simulink model "qpsk_rx_frame_sync"  (R2020a)
settings: Solver=VariableStepAuto  StartTime=0.0  StopTime=4000/3.2e6  RelTol=1e-3
PreLoadFcn:
  | setup_qpsk_receiver
InitFcn:
  | setup_qpsk_receiver
values from neighbouring files (symbols this model uses):
  tx_data = [tx_data mbuf]    [setup_receiver.m]
undefined symbols (not defined in the file or in its folder): AXI4, designMultirateFIR, Lite, xlfda_numerator
libraries: xbsIndex_r4 x244, dspmlti4 x11, hdlsllib x9, dspswit3 x4, commrandsrc3 x2, dspsigops x2, simulink x1
(part 2 of 4)

== system qpsk_rx_frame_sync/QPSK System/QPSK RX Generation ==
  Data In : Inport
  CIC Decimation : dspmlti4/CIC Decimation  filtFrom=Dialog parameters  filtobj=CICDECIM  ftype=Decimator  R=5  M=1  N=3  filterInternals=Full precision  BPS=[16 16 16 16]  FLPS=0  outputWordLength=32  outputFracLength=0  launchFVT=off  framing=Maintain input frame rate  RateOptions=Allow multirate processing
      settings: SourceProductBaseCode=DS
  FDATool : xbsIndex_r4/FDATool  block_type=fdatool
      settings: infoedit=FDATool
  FIR 0 : dspmlti4/FIR Decimation  FilterSource=Dialog parameters  h=xlfda_numerator('FDATool')  D=2  filtStruct=Direct form  FilterObject=fir0  framing=Enforce single-rate processing  inputOffset=0  outputBufInitCond=0  roundingMode=Floor  overflowMode=off  firstCoeffDataTypeStr=Inherit: Same word length as input  firstCoeffMin=[]  firstCoeffMax=[]  firstCoeffLastDataTypeStr=Inherit: Same word length as input  outputMode=Binary point scaling  outputWordLength=16  outputFracLength=14  outputDataTypeStr=fixdt(1,16,14)  outputMin=[]  outputMax=[]  outputLastDataTypeStr=fixdt(1,16,14)
  Gain : Gain  Gain=2^(floor(log2(5^3)))/(5^3)  ParamDataTypeStr=fixdt(1,16,14)  OutDataTypeStr=fixdt(1,16,14)
  RRC Receive Filter : Subsystem
  Shift Arithmetic : ArithShift  BitShiftNumber=floor(log2(5^3))  BitShiftDirection=Right
  Unbuffer : Unbuffer
  Data Out : Outport  VectorParamsAs1DForOutWhenUnconnected=off
  wires:
  RRC Receive Filter/1(Data Out) -> Data Out/1
  Gain/1 -> RRC Receive Filter/1(Data In)
  Shift Arithmetic/1 -> Gain/1
  CIC Decimation/1 -> Shift Arithmetic/1
  FIR 0/1 -> CIC Decimation/1
  Data In/1 -> Unbuffer/1
  Unbuffer/1 -> FIR 0/1

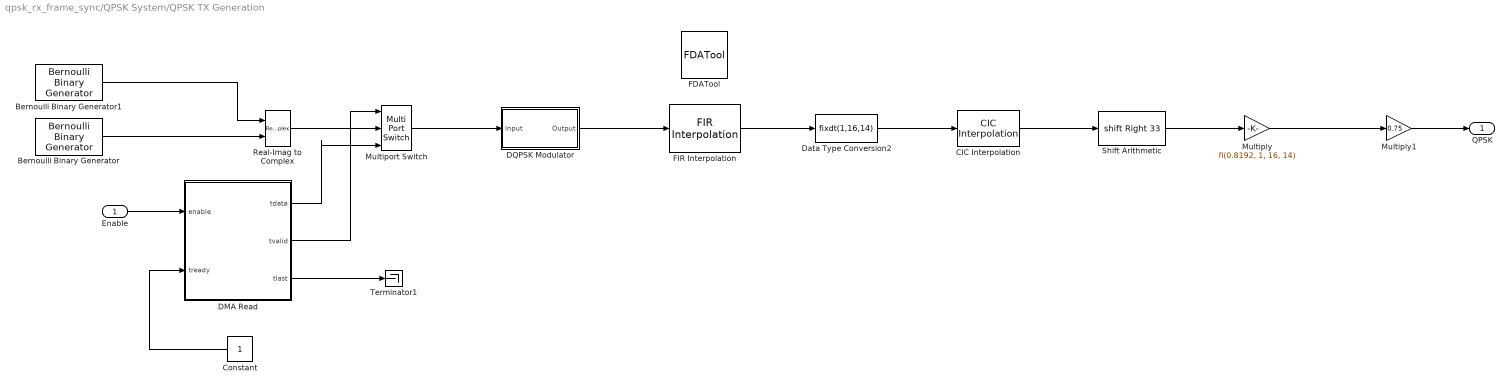
== system qpsk_rx_frame_sync/QPSK System/QPSK TX Generation ==
  Enable : Inport
  Bernoulli Binary Generator : commrandsrc3/Bernoulli Binary Generator  ProbabilityOfZero=0.5  SeedSource=Parameter  Seed=53  SampleTime=1/100e3  SamplesPerFrame=1  OutputDataType=double  SimulateUsing=Interpreted execution
  Bernoulli Binary Generator1 : commrandsrc3/Bernoulli Binary Generator  ProbabilityOfZero=0.5  SeedSource=Parameter  Seed=1  SampleTime=1/100e3  SamplesPerFrame=1  OutputDataType=double  SimulateUsing=Interpreted execution
  CIC Interpolation : dspmlti4/CIC Interpolation  filtFrom=Dialog parameters  filtobj=Hm_interp  ftype=Interpolator  R=320  M=1  N=5  filterInternals=Full precision  BPS=[16 16 16 16]  FLPS=0  outputWordLength=32  outputFracLength=0  launchFVT=off  framing=Allow multirate processing  OutputFrames=off
      settings: SourceProductBaseCode=DS
  Constant : Constant  SampleTime=1/25e3
  DMA Read : Subsystem
  DQPSK Modulator : Subsystem
  Data Type Conversion2 : DataTypeConversion  OutDataTypeStr=fixdt(1,16,14)
  FDATool : xbsIndex_r4/FDATool  block_type=fdatool
      settings: infoedit=FDATool
  FIR Interpolation : dspmlti4/FIR Interpolation  FilterSource=Dialog parameters  PrivateCoeffs=0  h=xlfda_numerator('FDATool')*4  L=4  FilterObject=xlfda_numerator('FDATool')/(max(xlfda_numerator('FDATool')))  framing=Allow multirate processing  outputBufInitCond=0  roundingMode=Floor  overflowMode=off  firstCoeffMode=Binary point scaling  firstCoeffWordLength=16  firstCoeffFracLength=14  firstCoeffDataTypeStr=fixdt(1,16,14)  firstCoeffMin=[]  firstCoeffMax=[]  firstCoeffLastDataTypeStr=fixdt(1,16,14)  outputDataTypeStr=Inherit: Same as accumulator  outputMin=[]  outputMax=[]  outputLastDataTypeStr=Inherit: Same as accumulator
  Multiply : Gain  Gain=fi(0.8192, 1, 16, 14)  ParamDataTypeStr=fixdt(1,16,15)  OutDataTypeStr=fixdt(1,16,14)
  Multiply1 : Gain  Gain=0.75  ParamDataTypeStr=double  OutDataTypeStr=fixdt(1,16,14)
  Multiport Switch : MultiPortSwitch  DataPortOrder=Zero-based contiguous  Inputs=2  zeroidx=on
  Real-Imag to Complex : RealImagToComplex
  Shift Arithmetic : ArithShift  BitShiftNumber=33  BitShiftDirection=Right
  Terminator1 : Terminator
  QPSK : Outport  VectorParamsAs1DForOutWhenUnconnected=off
  wires:
  Real-Imag to Complex/1 -> Multiport Switch/2
  Bernoulli Binary Generator/1 -> Real-Imag to Complex/2
  Bernoulli Binary Generator1/1 -> Real-Imag to Complex/1
  CIC Interpolation/1 -> Shift Arithmetic/1
  FIR Interpolation/1 -> Data Type Conversion2/1
  DMA Read/2(tvalid) -> Multiport Switch/1
  DMA Read/1(tdata) -> Multiport Switch/3
  DMA Read/3(tlast) -> Terminator1/1
  Enable/1 -> DMA Read/1(enable)
  Constant/1 -> DMA Read/2(tready)
  Multiport Switch/1 -> DQPSK Modulator/1(Input)
  DQPSK Modulator/1(Output) -> FIR Interpolation/1
  Data Type Conversion2/1 -> CIC Interpolation/1
  Shift Arithmetic/1 -> Multiply/1
  Multiply/1 -> Multiply1/1
  Multiply1/1 -> QPSK/1

== system qpsk_rx_frame_sync/QPSK System/RF-ADC ==
  Data In : Inport
  Decimation Filter : Subsystem  mask{decim=8x}
      mask prompts: decim "Decimation Factor:"
      mask init:
      | fir0 = dsp.FIRDecimator('DecimationFactor', 2,...
      |                            'CoefficientsDataType', 'Custom',...
      |                            'CustomCoefficientsDataType', numerictype([], 16, 14),...
      |                            'FullPrecisionOverride', false,...
      |                            'OutputDataType', 'Custom',...
      |                            'CustomOutputDataType', numerictype([], 16, 14),...
      |                            'Numerator', [-6, 0 54, 0, -254, 0, 1230, 2048, 1230, 0, -254, 0, 54, 0, -6]/(2048*2));
      | fir1 = dsp.FIRDecimator('DecimationFactor', 2,...
      |                            'CoefficientsDataType', 'Custom',...
      |                            'CustomCoefficientsDataType', numerictype([], 16, 14),...
      |                            'FullPrecisionOverride', false,...
      |                            'OutputDataType', 'Custom',...
      |                            'CustomOutputDataType', numerictype([], 16, 14),...
      |                            'Numerator', [-12, 0, 84, 0, -337, 0, 1008, 0, -2693, 0, 10142, 16384, 10142, 0, -2693, 0, 1008, 0, -337, 0, 84, 0 ,-12]/(16384*2));
      | fir2 = dsp.FIRDecimator('DecimationFactor', 2,...
      |                            'CoefficientsDataType', 'Custom',...
      |                            'CustomCoefficientsDataType', numerictype([], 16, 14),...
      |                            'FullPrecisionOverride', false,...
      |                            'OutputDataType', 'Custom',...
      |                            'CustomOutputDataType', numerictype([], 16, 14),...
      |                            'Numerator', [5, 0, -17, 0, 44, 0, -96, 0, 187, 0, -335, 0, 565, 0, -906, 0, 1401, 0, -2112, 0, 3145, 0, -4723, 0, 7415, 0, -13331, 0, 41526, 65536, 41526, 0, -13331, 0, 7415, 0, -4723, 0, 3145, 0, -2112, 0, 1401, 0, -906, 0, 565, 0, -335, 0, 187, 0, -96, 0, 44, 0, -17, 0, 5]/(65536*2));
      | switch get_param(gcb, 'decim')
      |     case '1x'
      |         if ~strcmp(get_param([gcb, '/FIR 0'], 'Commented'), 'through')
      |             set_param([gcb, '/FIR 0'],'Commented','through');
      |         end
      |         
      |         if ~strcmp(get_param([gcb, '/FIR 1'], 'Commented'), 'through')
      |             set_param([gcb, '/FIR 1'],'Commented','through');
      |         end
      |         
      |         if ~strcmp(get_param([gcb, '/FIR 2'], 'Commented'), 'through')
      |             set_param([gcb, '/FIR 2'],'Commented','through');
      |         end
      |             
      |     case '2x'
      |         if ~strcmp(get_param([gcb, '/FIR 0'], 'Commented'), 'through')
      |             set_param([gcb, '/FIR 0'],'Commented','through');
      |         end
      |         
      |         if ~strcmp(get_param([gcb, '/FIR 1'], 'Commented'), 'through')
      |             set_param([gcb, '/FIR 1'],'Commented','through');
      |         end
      |         
      |         if ~strcmp(get_param([gcb, '/FIR 2'], 'Commented'), 'off')
      |             set_param([gcb, '/FIR 2'],'Commented','off');
      |         end
      | 
      |     case '4x'
      |         if ~strcmp(get_param([gcb, '/FIR 0'], 'Commented'), 'through')
      |             set_param([gcb, '/FIR 0'],'Commented','through');
      |         end
      |         
      |         if ~strcmp(get_param([gcb, '/FIR 1'], 'Commented'), 'off')
      |             set_param([gcb, '/FIR 1'],'Commented','off');
      |         end
      |         
      |         if ~strcmp(get_param([gcb, '/FIR 2'], 'Commented'), 'off')
      |             set_param([gcb, '/FIR 2'],'Commented','off');
      |         end
      |         
      |     case '8x'
      |         if ~strcmp(get_param([gcb, '/FIR 0'], 'Commented'), 'off')
      |             set_param([gcb, '/FIR 0'],'Commented','off');
      |         end
      |         
      |         if ~strcmp(get_param([gcb, '/FIR 1'], 'Commented'), 'off')
      |             set_param([gcb, '/FIR 1'],'Commented','off');
      |         end
      |         
      |         if ~strcmp(get_param([gcb, '/FIR 2'], 'Commented'), 'off')
      |             set_param([gcb, '/FIR 2'],'Commented','off');
      |         end
      | 
      | end
      mask TypeOptions decim: 1x | 2x | 4x | 8x
      mask DialogControl DescGroupVar Prompt: RF-DAC Interpolation Filter
      mask DialogControl DescTextVar Prompt: This block simulates the RF-DAC interpolation stage using the same coefficients stored in the interpolation filters.
      mask DialogControl ParameterGroupVar Prompt: Main
  NCO and Mixer : Subsystem
  RF-ADC : Subsystem
  Data Out : Outport  VectorParamsAs1DForOutWhenUnconnected=off
  wires:
  RF-ADC/1(Data Out) -> NCO and Mixer/1(Data In)
  Data In/1 -> RF-ADC/1(Data In)
  Decimation Filter/1(Data Out) -> Data Out/1
  NCO and Mixer/1(Data Out) -> Decimation Filter/1(Data In)

== system qpsk_rx_frame_sync/QPSK System/RF-DAC ==
  note: Not Ready
  Data In : Inport
  Coarse Delay : Subsystem
  Interpolation Filter : Subsystem  mask{interp=8x}
      mask prompts: interp "Interpolation Factor:"
      mask init:
      | fir0 = dsp.FIRInterpolator('InterpolationFactor', 2,...
      |                            'CoefficientsDataType', 'Custom',...
      |                            'CustomCoefficientsDataType', numerictype([], 16, 14),...
      |                            'FullPrecisionOverride', false,...
      |                            'OutputDataType', 'Custom',...
      |                            'CustomOutputDataType', numerictype([], 16, 14),...
      |                            'Numerator', [-6, 0 54, 0, -254, 0, 1230, 2048, 1230, 0, -254, 0, 54, 0, -6]/(2048));
      | fir1 = dsp.FIRInterpolator('InterpolationFactor', 2,...
      |                            'CoefficientsDataType', 'Custom',...
      |                            'CustomCoefficientsDataType', numerictype([], 16, 14),...
      |                            'FullPrecisionOverride', false,...
      |                            'OutputDataType', 'Custom',...
      |                            'CustomOutputDataType', numerictype([], 16, 14),...
      |                            'Numerator', [-12, 0, 84, 0, -337, 0, 1008, 0, -2693, 0, 10142, 16384, 10142, 0, -2693, 0, 1008, 0, -337, 0, 84, 0 ,-12]/(16384));
      | fir2 = dsp.FIRInterpolator('InterpolationFactor', 2,...
      |                            'CoefficientsDataType', 'Custom',...
      |                            'CustomCoefficientsDataType', numerictype([], 16, 14),...
      |                            'FullPrecisionOverride', false,...
      |                            'OutputDataType', 'Custom',...
      |                            'CustomOutputDataType', numerictype([], 16, 14),...
      |                            'Numerator', [5, 0, -17, 0, 44, 0, -96, 0, 187, 0, -335, 0, 565, 0, -906, 0, 1401, 0, -2112, 0, 3145, 0, -4723, 0, 7415, 0, -13331, 0, 41526, 65536, 41526, 0, -13331, 0, 7415, 0, -4723, 0, 3145, 0, -2112, 0, 1401, 0, -906, 0, 565, 0, -335, 0, 187, 0, -96, 0, 44, 0, -17, 0, 5]/(65536));
      | switch get_param(gcb, 'interp')
      |     case '1x'
      |         if ~strcmp(get_param([gcb, '/FIR 0'], 'Commented'), 'through')
      |             set_param([gcb, '/FIR 0'],'Commented','through');
      |         end
      |         
      |         if ~strcmp(get_param([gcb, '/FIR 1'], 'Commented'), 'through')
      |             set_param([gcb, '/FIR 1'],'Commented','through');
      |         end
      |         
      |         if ~strcmp(get_param([gcb, '/FIR 2'], 'Commented'), 'through')
      |             set_param([gcb, '/FIR 2'],'Commented','through');
      |         end
      |             
      |     case '2x'
      |         if ~strcmp(get_param([gcb, '/FIR 0'], 'Commented'), 'through')
      |             set_param([gcb, '/FIR 0'],'Commented','through');
      |         end
      |         
      |         if ~strcmp(get_param([gcb, '/FIR 1'], 'Commented'), 'through')
      |             set_param([gcb, '/FIR 1'],'Commented','through');
      |         end
      |         
      |         if ~strcmp(get_param([gcb, '/FIR 2'], 'Commented'), 'off')
      |             set_param([gcb, '/FIR 2'],'Commented','off');
      |         end
      | 
      |     case '4x'
      |         if ~strcmp(get_param([gcb, '/FIR 0'], 'Commented'), 'through')
      |             set_param([gcb, '/FIR 0'],'Commented','through');
      |         end
      |         
      |         if ~strcmp(get_param([gcb, '/FIR 1'], 'Commented'), 'off')
      |             set_param([gcb, '/FIR 1'],'Commented','off');
      |         end
      |         
      |         if ~strcmp(get_param([gcb, '/FIR 2'], 'Commented'), 'off')
      |             set_param([gcb, '/FIR 2'],'Commented','off');
      |         end
      |         
      |     case '8x'
      |         if ~strcmp(get_param([gcb, '/FIR 0'], 'Commented'), 'off')
      |             set_param([gcb, '/FIR 0'],'Commented','off');
      |         end
      |         
      |         if ~strcmp(get_param([gcb, '/FIR 1'], 'Commented'), 'off')
      |             set_param([gcb, '/FIR 1'],'Commented','off');
      |         end
      |         
      |         if ~strcmp(get_param([gcb, '/FIR 2'], 'Commented'), 'off')
      |             set_param([gcb, '/FIR 2'],'Commented','off');
      |         end
      | 
      | end
      mask TypeOptions interp: 1x | 2x | 4x | 8x
      mask DialogControl DescGroupVar Prompt: RF-DAC Interpolation Filter
      mask DialogControl DescTextVar Prompt: This block simulates the RF-DAC interpolation stage using the same coefficients stored in the interpolation filters.
      mask DialogControl ParameterGroupVar Prompt: Main
  NCO and Mixer : Subsystem
  Output Filter : Subsystem
  QMC Gain & Phase : Subsystem
  QMC Threshold : Subsystem
  RF-DAC : Subsystem
  Data Out : Outport  VectorParamsAs1DForOutWhenUnconnected=off
  wires:
  RF-DAC/1(Data Out) -> Data Out/1
  QMC Threshold/1(Data Out) -> RF-DAC/1(Data In)
  Output Filter/1(Data Out) -> QMC Threshold/1(Data In)
  Coarse Delay/1(Data Out) -> Output Filter/1(Data In)
  QMC Gain & Phase/1(Data Out) -> Coarse Delay/1(Data In)
  Data In/1 -> Interpolation Filter/1(Data In)
  NCO and Mixer/1(Data Out) -> QMC Gain & Phase/1(Data In)
  Interpolation Filter/1(Data Out) -> NCO and Mixer/1(Data In)

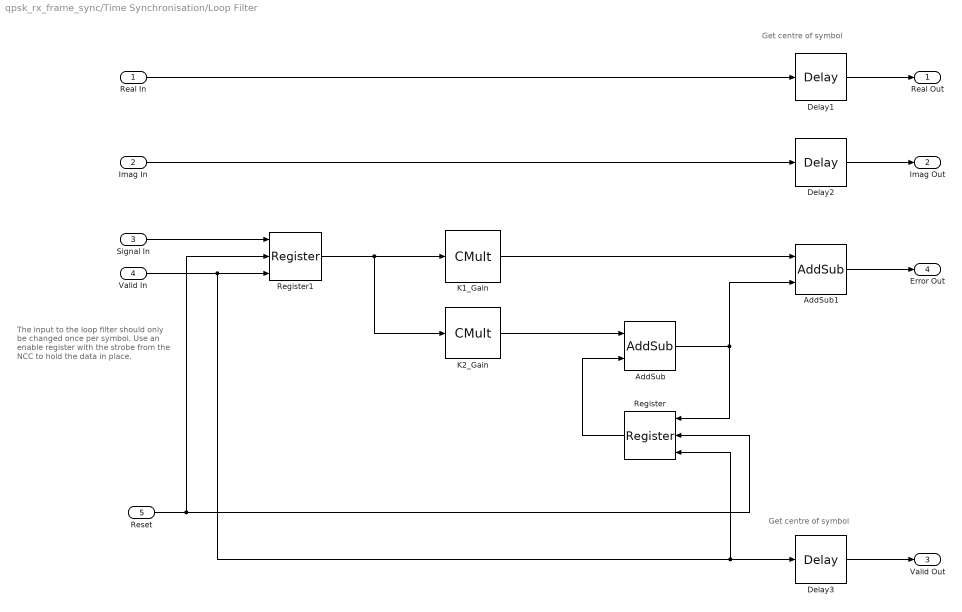
== system qpsk_rx_frame_sync/Time Synchronisation/Loop Filter ==
  note: Get centre of symbol
  note: The input to the loop filter should only be changed once per symbol.
      |
      | Use an enable register with the strobe from the NCC to hold the data in place.
  note: Get centre of symbol
  Real In : Inport
  Imag In : Inport  Port=2
  Signal In : Inport  Port=3
  Valid In : Inport  Port=4
  Reset : Inport  Port=5
  AddSub : xbsIndex_r4/AddSub  mode=Addition  use_carryin=off  use_carryout=off  en=off  latency=0  precision=User Defined  arith_type="Signed  (2's comp)"  n_bits=52  bin_pt=44  quantization=Truncate  overflow=Flag as error  use_behavioral_HDL=off  hw_selection=Fabric  pipelined=off  dbl_ovrd=off  block_type=addsub
  AddSub1 : xbsIndex_r4/AddSub  mode=Addition  use_carryin=off  use_carryout=off  en=off  latency=0  precision=Full  arith_type="Signed  (2's comp)"  n_bits=32  bin_pt=31  quantization=Truncate  overflow=Wrap  use_behavioral_HDL=off  hw_selection=Fabric  pipelined=off  dbl_ovrd=off  block_type=addsub
  Delay1 : xbsIndex_r4/Delay  rst=off  infoeditControl=Selection of Reset will increase slice count due to use of real FFs and instead of SRLs  en=off  latency=32/2  reg_retiming=off  dbl_ovrd=off  block_type=delay
  Delay2 : xbsIndex_r4/Delay  rst=off  infoeditControl=Selection of Reset will increase slice count due to use of real FFs and instead of SRLs  en=off  latency=32/2  reg_retiming=off  dbl_ovrd=off  block_type=delay
  Delay3 : xbsIndex_r4/Delay  rst=off  infoeditControl=Selection of Reset will increase slice count due to use of real FFs and instead of SRLs  en=off  latency=32/2  reg_retiming=off  dbl_ovrd=off  block_type=delay
  K1_Gain : xbsIndex_r4/CMult  const=K1  gui_display_data_type=Fixed-point  const_n_bits=18  const_bin_pt=16  float_type=Single  exp_bits=8  fraction_bits=24  en=off  latency=0  precision=Full  arith_type="Signed  (2's comp)"  n_bits=3+28+16  bin_pt=28+16  quantization=Truncate  overflow=Wrap  use_behavioral_HDL=off  mem_type=Distributed RAM  pipeline=off  dbl_ovrd=off  block_type=cmult
  K2_Gain : xbsIndex_r4/CMult  const=K2  gui_display_data_type=Fixed-point  const_n_bits=18  const_bin_pt=16  float_type=Single  exp_bits=8  fraction_bits=24  en=off  latency=0  precision=Full  arith_type="Signed  (2's comp)"  n_bits=3+28+16  bin_pt=28+16  quantization=Truncate  overflow=Wrap  use_behavioral_HDL=off  mem_type=Distributed RAM  pipeline=off  dbl_ovrd=off  block_type=cmult
  Register : xbsIndex_r4/Register  init=0  rst=on  en=on  dbl_ovrd=off  block_type=register
  Register1 : xbsIndex_r4/Register  init=0  rst=on  en=on  dbl_ovrd=off  block_type=register
  Real Out : Outport  VectorParamsAs1DForOutWhenUnconnected=off
  Imag Out : Outport  Port=2  VectorParamsAs1DForOutWhenUnconnected=off
  Valid Out : Outport  Port=3  VectorParamsAs1DForOutWhenUnconnected=off
  Error Out : Outport  Port=4  VectorParamsAs1DForOutWhenUnconnected=off
  wires:
  Delay3/1 -> Valid Out/1
  Reset/1 -> Register/2, Register1/2
  K2_Gain/1 -> AddSub/1
  AddSub1/1 -> Error Out/1
  Real In/1 -> Delay1/1
  Imag In/1 -> Delay2/1
  AddSub/1 -> Register/1, AddSub1/2
  K1_Gain/1 -> AddSub1/1
  Register/1 -> AddSub/2
  Signal In/1 -> Register1/1
  Register1/1 -> K1_Gain/1, K2_Gain/1
  Delay2/1 -> Imag Out/1
  Delay1/1 -> Real Out/1
  Valid In/1 -> Delay3/1, Register/3, Register1/3

== system qpsk_rx_frame_sync/Time Synchronisation/NCC ==
  note: For the Numerically Controlled Clock (NCC), we need to consider
      | the symbol oversample factor and the fractional wordlength
      | of the accumulator.
      |
      | The number of samples per symbol determine the maximum value
      | of the accumulator {ceil(log2(n))+1}.
      |
      | The fractional bits determine the quantisation step (precision),
      | of our accumulator.
      |
      | We add 1 to the error signal at all times, as this is necessary to
      | ensure the accumulator always adds 1. If the error is equal to
      | zero, then the accumulator will increase normally. If there is an
      | error in phase not equal to zero, the accumulator will change to
      | compensate for the phase difference.
  Error : Inport
  AddSub : xbsIndex_r4/AddSub  mode=Addition  use_carryin=off  use_carryout=off  en=off  latency=0  precision=User Defined  arith_type=Unsigned  n_bits=n+44  bin_pt=44  quantization=Truncate  overflow=Wrap  use_behavioral_HDL=off  hw_selection=Fabric  pipelined=off  dbl_ovrd=off  block_type=addsub
  AddSub1 : xbsIndex_r4/AddSub  mode=Addition  use_carryin=off  use_carryout=off  en=off  latency=0  precision=Full  arith_type="Signed  (2's comp)"  n_bits=45  bin_pt=44  quantization=Truncate  overflow=Flag as error  use_behavioral_HDL=off  hw_selection=Fabric  pipelined=off  dbl_ovrd=off  block_type=addsub
  Constant : xbsIndex_r4/Constant  const=1  gui_display_data_type=Fixed-point  arith_type=Unsigned  n_bits=1  bin_pt=0  preci_type=Single  exp_width=8  frac_width=24  explicit_period=off  period=1  equ=P=C  opselect=C  inp2=PCIN>>17  opr=+  inp1=P  carry=CIN  dbl_ovrd=off  block_type=constant
  Register : xbsIndex_r4/Register  init=0  rst=off  en=off  dbl_ovrd=off  block_type=register
  Relational : xbsIndex_r4/Relational  mode=a<b  op_type=Bool  en=off  latency=0  dbl_ovrd=off  block_type=relational
  Strobe : Outport  VectorParamsAs1DForOutWhenUnconnected=off
  wires:
  Register/1 -> AddSub/1, Relational/2
  Relational/1 -> Strobe/1
  AddSub/1 -> Register/1, Relational/1
  AddSub1/1 -> AddSub/2
  Constant/1 -> AddSub1/1
  Error/1 -> AddSub1/2

== system qpsk_rx_frame_sync/Time Synchronisation/Timing Error Detector ==
  Real In : Inport
  Imag In : Inport  Port=2
  AddSub : xbsIndex_r4/AddSub  mode=Subtraction  use_carryin=off  use_carryout=off  en=off  latency=0  precision=Full  arith_type=Unsigned  n_bits=16  bin_pt=14  quantization=Truncate  overflow=Wrap  use_behavioral_HDL=off  hw_selection=Fabric  pipelined=off  dbl_ovrd=off  block_type=addsub
  AddSub1 : xbsIndex_r4/AddSub  mode=Subtraction  use_carryin=off  use_carryout=off  en=off  latency=0  precision=Full  arith_type=Unsigned  n_bits=16  bin_pt=14  quantization=Truncate  overflow=Wrap  use_behavioral_HDL=off  hw_selection=Fabric  pipelined=off  dbl_ovrd=off  block_type=addsub
  AddSub2 : xbsIndex_r4/AddSub  mode=Addition  use_carryin=off  use_carryout=off  en=off  latency=0  precision=Full  arith_type="Signed  (2's comp)"  n_bits=33  bin_pt=25  quantization="Round  (unbiased: +/- Inf)"  overflow=Saturate  use_behavioral_HDL=off  hw_selection=Fabric  pipelined=off  dbl_ovrd=off  block_type=addsub
  Delay : xbsIndex_r4/Delay  rst=off  infoeditControl=Selection of Reset will increase slice count due to use of real FFs and instead of SRLs  en=off  latency=32  reg_retiming=off  dbl_ovrd=off  block_type=delay
  Delay1 : xbsIndex_r4/Delay  rst=off  infoeditControl=Selection of Reset will increase slice count due to use of real FFs and instead of SRLs  en=off  latency=32  reg_retiming=off  dbl_ovrd=off  block_type=delay
  Mult1 : xbsIndex_r4/Mult  precision=Full  arith_type=Unsigned  n_bits=31  bin_pt=28  quantization=Truncate  overflow=Saturate  en=off  latency=0  use_behavioral_HDL=off  opt=Speed  use_embedded=on  optimum_pipeline=off  pipeline=on  dbl_ovrd=off  use_rpm=on  placement_style=Triangular  block_type=mult
  Mult2 : xbsIndex_r4/Mult  precision=Full  arith_type=Unsigned  n_bits=31  bin_pt=28  quantization=Truncate  overflow=Saturate  en=off  latency=0  use_behavioral_HDL=off  opt=Speed  use_embedded=on  optimum_pipeline=off  pipeline=on  dbl_ovrd=off  use_rpm=on  placement_style=Triangular  block_type=mult
  Error : Outport  VectorParamsAs1DForOutWhenUnconnected=off
  wires:
  Real In/1 -> Mult1/1, Mult1/2
  Imag In/1 -> Mult2/1, Mult2/2
  AddSub/1 -> AddSub2/1
  AddSub2/1 -> Error/1
  Delay1/1 -> AddSub1/2
  Mult2/1 -> Delay1/1, AddSub1/1
  AddSub1/1 -> AddSub2/2
  Mult1/1 -> AddSub/1, Delay/1
  Delay/1 -> AddSub/2

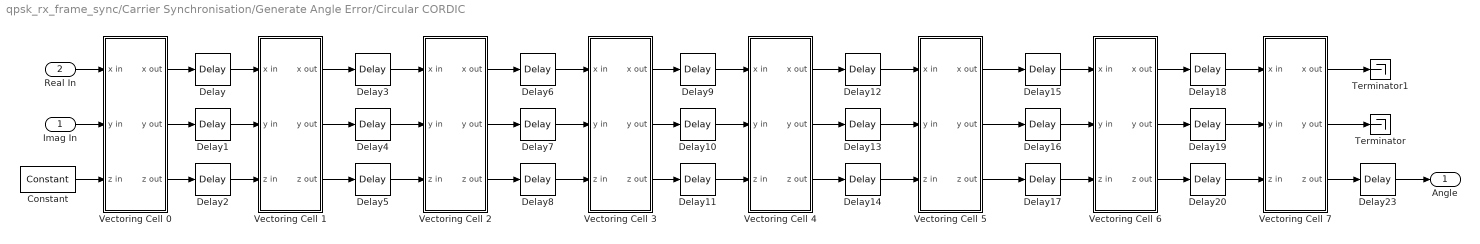
== system qpsk_rx_frame_sync/Carrier Synchronisation/Generate Angle Error/Circular CORDIC ==
  Imag In : Inport
  Real In : Inport  Port=2
  Constant : xbsIndex_r4/Constant  const=0  gui_display_data_type=Fixed-point  arith_type=Signed (2's comp)  n_bits=16  bin_pt=14  preci_type=Single  exp_width=8  frac_width=24  explicit_period=off  period=1  equ=P=C  opselect=C  inp2=PCIN>>17  opr=+  inp1=P  carry=CIN  dbl_ovrd=off  block_type=constant
  Delay{,1..20,23} (22 alike) : xbsIndex_r4/Delay  rst=off  infoeditControl=Selection of Reset will increase slice count due to use of real FFs and instead of SRLs  en=off  latency=1  reg_retiming=off  dbl_ovrd=off  block_type=delay
  Terminator : Terminator
  Terminator1 : Terminator
  Vectoring Cell 0 : Subsystem  mask(Cordic Vectoring Cell){i=0}
      mask prompts: i "Iteration:"
      mask help: some notes to go here
      mask DialogControl DescGroupVar Prompt: CORDIC Vectoring Cell
      mask DialogControl DescTextVar Prompt: A single cell of a vectoring CORDIC unrolled architecture.
      mask DialogControl ParameterGroupVar Prompt: Main
  Vectoring Cell 1 : Subsystem  mask(Cordic Vectoring Cell){i=1}
      mask prompts: i "Iteration:"
      mask help: some notes to go here
      mask DialogControl DescGroupVar Prompt: CORDIC Vectoring Cell
      mask DialogControl DescTextVar Prompt: A single cell of a vectoring CORDIC unrolled architecture.
      mask DialogControl ParameterGroupVar Prompt: Main
  Vectoring Cell 2 : Subsystem  mask(Cordic Vectoring Cell){i=2}
      mask prompts: i "Iteration:"
      mask help: some notes to go here
      mask DialogControl DescGroupVar Prompt: CORDIC Vectoring Cell
      mask DialogControl DescTextVar Prompt: A single cell of a vectoring CORDIC unrolled architecture.
      mask DialogControl ParameterGroupVar Prompt: Main
  Vectoring Cell 3 : Subsystem  mask(Cordic Vectoring Cell){i=3}
      mask prompts: i "Iteration:"
      mask help: some notes to go here
      mask DialogControl DescGroupVar Prompt: CORDIC Vectoring Cell
      mask DialogControl DescTextVar Prompt: A single cell of a vectoring CORDIC unrolled architecture.
      mask DialogControl ParameterGroupVar Prompt: Main
  Vectoring Cell 4 : Subsystem  mask(Cordic Vectoring Cell){i=4}
      mask prompts: i "Iteration:"
      mask help: some notes to go here
      mask DialogControl DescGroupVar Prompt: CORDIC Vectoring Cell
      mask DialogControl DescTextVar Prompt: A single cell of a vectoring CORDIC unrolled architecture.
      mask DialogControl ParameterGroupVar Prompt: Main
  Vectoring Cell 5 : Subsystem  mask(Cordic Vectoring Cell){i=5}
      mask prompts: i "Iteration:"
      mask help: some notes to go here
      mask DialogControl DescGroupVar Prompt: CORDIC Vectoring Cell
      mask DialogControl DescTextVar Prompt: A single cell of a vectoring CORDIC unrolled architecture.
      mask DialogControl ParameterGroupVar Prompt: Main
  Vectoring Cell 6 : Subsystem  mask(Cordic Vectoring Cell){i=6}
      mask prompts: i "Iteration:"
      mask help: some notes to go here
      mask DialogControl DescGroupVar Prompt: CORDIC Vectoring Cell
      mask DialogControl DescTextVar Prompt: A single cell of a vectoring CORDIC unrolled architecture.
      mask DialogControl ParameterGroupVar Prompt: Main
  Vectoring Cell 7 : Subsystem  mask(Cordic Vectoring Cell){i=7}
      mask prompts: i "Iteration:"
      mask help: some notes to go here
      mask DialogControl DescGroupVar Prompt: CORDIC Vectoring Cell
      mask DialogControl DescTextVar Prompt: A single cell of a vectoring CORDIC unrolled architecture.
      mask DialogControl ParameterGroupVar Prompt: Main
  Angle : Outport  VectorParamsAs1DForOutWhenUnconnected=off
  wires:
  Vectoring Cell 6/3(z out) -> Delay20/1
  Delay5/1 -> Vectoring Cell 2/3(z in)
  Vectoring Cell 6/2(y out) -> Delay19/1
  Vectoring Cell 2/1(x out) -> Delay6/1
  Vectoring Cell 1/3(z out) -> Delay5/1
  Delay14/1 -> Vectoring Cell 5/3(z in)
  Delay20/1 -> Vectoring Cell 7/3(z in)
  Delay15/1 -> Vectoring Cell 6/1(x in)
  Delay7/1 -> Vectoring Cell 3/2(y in)
  Delay1/1 -> Vectoring Cell 1/2(y in)
  Vectoring Cell 3/1(x out) -> Delay9/1
  Delay13/1 -> Vectoring Cell 5/2(y in)
  Delay9/1 -> Vectoring Cell 4/1(x in)
  Vectoring Cell 1/1(x out) -> Delay3/1
  Delay16/1 -> Vectoring Cell 6/2(y in)
  Delay18/1 -> Vectoring Cell 7/1(x in)
  Vectoring Cell 0/3(z out) -> Delay2/1
  Delay10/1 -> Vectoring Cell 4/2(y in)
  Vectoring Cell 2/2(y out) -> Delay7/1
  Vectoring Cell 3/3(z out) -> Delay11/1
  Delay6/1 -> Vectoring Cell 3/1(x in)
  Delay19/1 -> Vectoring Cell 7/2(y in)
  Delay4/1 -> Vectoring Cell 2/2(y in)
  Delay3/1 -> Vectoring Cell 2/1(x in)
  Vectoring Cell 4/3(z out) -> Delay14/1
  Delay8/1 -> Vectoring Cell 3/3(z in)
  Vectoring Cell 3/2(y out) -> Delay10/1
  Vectoring Cell 1/2(y out) -> Delay4/1
  Vectoring Cell 5/1(x out) -> Delay15/1
  Delay/1 -> Vectoring Cell 1/1(x in)
  Vectoring Cell 5/2(y out) -> Delay16/1
  Vectoring Cell 0/1(x out) -> Delay/1
  Vectoring Cell 2/3(z out) -> Delay8/1
  Vectoring Cell 6/1(x out) -> Delay18/1
  Vectoring Cell 0/2(y out) -> Delay1/1
  Delay12/1 -> Vectoring Cell 5/1(x in)
  Vectoring Cell 4/2(y out) -> Delay13/1
  Vectoring Cell 4/1(x out) -> Delay12/1
  Delay2/1 -> Vectoring Cell 1/3(z in)
  Vectoring Cell 5/3(z out) -> Delay17/1
  Delay17/1 -> Vectoring Cell 6/3(z in)
  Delay11/1 -> Vectoring Cell 4/3(z in)
  Vectoring Cell 7/3(z out) -> Delay23/1
  Real In/1 -> Vectoring Cell 0/1(x in)
  Imag In/1 -> Vectoring Cell 0/2(y in)
  Constant/1 -> Vectoring Cell 0/3(z in)
  Delay23/1 -> Angle/1
  Vectoring Cell 7/2(y out) -> Terminator/1
  Vectoring Cell 7/1(x out) -> Terminator1/1

== system qpsk_rx_frame_sync/Carrier Synchronisation/Generate NCO/Loop Filter ==
  Signal : Inport
  Strobe : Inport  Port=2
  Reset : Inport  Port=3
  AddSub : xbsIndex_r4/AddSub  mode=Addition  use_carryin=off  use_carryout=off  en=off  latency=0  precision=User Defined  arith_type="Signed  (2's comp)"  n_bits=36  bin_pt=34  quantization=Truncate  overflow=Flag as error  use_behavioral_HDL=off  hw_selection=Fabric  pipelined=off  dbl_ovrd=off  block_type=addsub
  AddSub1 : xbsIndex_r4/AddSub  mode=Addition  use_carryin=off  use_carryout=off  en=off  latency=0  precision=Full  arith_type="Signed  (2's comp)"  n_bits=32  bin_pt=31  quantization=Truncate  overflow=Wrap  use_behavioral_HDL=off  hw_selection=Fabric  pipelined=off  dbl_ovrd=off  block_type=addsub
  K1_Gain : xbsIndex_r4/CMult  const=K1  gui_display_data_type=Fixed-point  const_n_bits=16  const_bin_pt=16  float_type=Single  exp_bits=8  fraction_bits=24  en=off  latency=0  precision=Full  arith_type="Signed  (2's comp)"  n_bits=20  bin_pt=14  quantization=Truncate  overflow=Wrap  use_behavioral_HDL=off  mem_type=Distributed RAM  pipeline=off  dbl_ovrd=off  block_type=cmult
  K2_Gain : xbsIndex_r4/CMult  const=K2  gui_display_data_type=Fixed-point  const_n_bits=16  const_bin_pt=16  float_type=Single  exp_bits=8  fraction_bits=24  en=off  latency=0  precision=Full  arith_type="Signed  (2's comp)"  n_bits=20  bin_pt=14  quantization=Truncate  overflow=Wrap  use_behavioral_HDL=off  mem_type=Distributed RAM  pipeline=off  dbl_ovrd=off  block_type=cmult
  Register : xbsIndex_r4/Register  init=0  rst=on  en=on  dbl_ovrd=off  block_type=register
  Register1 : xbsIndex_r4/Register  init=0  rst=on  en=on  dbl_ovrd=off  block_type=register
  Register3 : xbsIndex_r4/Register  init=0  rst=off  en=off  dbl_ovrd=off  block_type=register
  Register4 : xbsIndex_r4/Register  init=0  rst=off  en=off  dbl_ovrd=off  block_type=register
  Error : Outport  VectorParamsAs1DForOutWhenUnconnected=off
  Valid : Outport  Port=2  VectorParamsAs1DForOutWhenUnconnected=off
  wires:
  Reset/1 -> Register/2, Register1/2
  Signal/1 -> Register1/1
  K2_Gain/1 -> AddSub/1
  AddSub/1 -> AddSub1/2, Register/1
  Register/1 -> AddSub/2
  Register1/1 -> K2_Gain/1, K1_Gain/1
  AddSub1/1 -> Register3/1
  K1_Gain/1 -> AddSub1/1
  Register3/1 -> Error/1
  Register4/1 -> Valid/1
  Strobe/1 -> Register4/1, Register/3, Register1/3

== system qpsk_rx_frame_sync/Carrier Synchronisation/Generate NCO/NCO ==
  Step Size : Inport
  En_in : Inport  Port=2
  AddSub4 : xbsIndex_r4/AddSub  mode=Addition  use_carryin=off  use_carryout=off  en=off  latency=0  precision=User Defined  arith_type="Signed  (2's comp)"  n_bits=n+b  bin_pt=b  quantization=Truncate  overflow=Wrap  use_behavioral_HDL=off  hw_selection=Fabric  pipelined=off  dbl_ovrd=off  block_type=addsub
  CMult1 : xbsIndex_r4/CMult  const=(2^n)/(2*pi)  gui_display_data_type=Fixed-point  const_n_bits=k_n+b  const_bin_pt=b  float_type=Single  exp_bits=8  fraction_bits=24  en=off  latency=0  precision=User Defined  arith_type="Signed  (2's comp)"  n_bits=n+b  bin_pt=b  quantization=Truncate  overflow=Wrap  use_behavioral_HDL=off  mem_type=Distributed RAM  pipeline=off  dbl_ovrd=off  block_type=cmult
  Convert1 : xbsIndex_r4/Convert  gui_display_data_type=Fixed-point  arith_type=Unsigned  n_bits=n  bin_pt=0  float_type=Single  exp_bits=8  fraction_bits=24  quantization=Truncate  overflow=Wrap  en=off  latency=0  pipeline=off  dbl_ovrd=off  block_type=convert
  Cos ROM : xbsIndex_r4/ROM  depth=2^n  initVector=cos(pi*(0:((2^n)-1))/(2^(n-1)))  distributed_mem=Block RAM  rst=off  init_reg=0  en=off  latency=1  gui_display_data_type=Fixed-point  arith_type="Signed  (2's comp)"  n_bits=16  bin_pt=14  preci_type=Single  exp_width=8  frac_width=24  optimize=Area  use_rpm=on  dbl_ovrd=off  simulation_type=fast_sim  block_type=sprom
  Neg Sin ROM : xbsIndex_r4/ROM  depth=2^n  initVector=-sin(pi*(0:((2^n)-1))/(2^(n-1)))  distributed_mem=Block RAM  rst=off  init_reg=0  en=off  latency=1  gui_display_data_type=Fixed-point  arith_type="Signed  (2's comp)"  n_bits=16  bin_pt=14  preci_type=Single  exp_width=8  frac_width=24  optimize=Area  use_rpm=on  dbl_ovrd=off  simulation_type=fast_sim  block_type=sprom
  Register : xbsIndex_r4/Register  init=0  rst=off  en=off  dbl_ovrd=off  block_type=register
  Register1 : xbsIndex_r4/Register  init=0  rst=off  en=on  dbl_ovrd=off  block_type=register
  Cos : Outport  VectorParamsAs1DForOutWhenUnconnected=off
  Neg Sin : Outport  Port=2  VectorParamsAs1DForOutWhenUnconnected=off
  En_out : Outport  Port=3  VectorParamsAs1DForOutWhenUnconnected=off
  wires:
  Convert1/1 -> Neg Sin ROM/1, Cos ROM/1
  AddSub4/1 -> Register1/1, Convert1/1
  Neg Sin ROM/1 -> Neg Sin/1
  Register1/1 -> AddSub4/2
  CMult1/1 -> AddSub4/1
  Step Size/1 -> CMult1/1
  En_in/1 -> Register/1, Register1/2
  Cos ROM/1 -> Cos/1
  Register/1 -> En_out/1

== system qpsk_rx_frame_sync/Frame Synchronisation/Frame Sync/DQPSK Imag Convert ==
  Data In : Inport
  Valid In : Inport  Port=2
  Constant : xbsIndex_r4/Constant  const=1.0  gui_display_data_type=Fixed-point  arith_type=Signed (2's comp)  n_bits=2  bin_pt=0  preci_type=Single  exp_width=8  frac_width=24  explicit_period=off  period=1  equ=P=C  opselect=C  inp2=PCIN>>17  opr=+  inp1=P  carry=CIN  dbl_ovrd=off  block_type=constant
  Constant1 : xbsIndex_r4/Constant  const=-1.0  gui_display_data_type=Fixed-point  arith_type=Signed (2's comp)  n_bits=2  bin_pt=0  preci_type=Single  exp_width=8  frac_width=24  explicit_period=off  period=1  equ=P=C  opselect=C  inp2=PCIN>>17  opr=+  inp1=P  carry=CIN  dbl_ovrd=off  block_type=constant
  Mux : xbsIndex_r4/Mux  inputs=2  en=off  latency=0  precision=Full  arith_type=Unsigned  n_bits=16  bin_pt=14  quantization=Truncate  overflow=Wrap  dbl_ovrd=off  block_type=mux
  Data Out : Outport  VectorParamsAs1DForOutWhenUnconnected=off
  Valid Out : Outport  Port=2  VectorParamsAs1DForOutWhenUnconnected=off
  wires:
  Data In/1 -> Mux/1
  Valid In/1 -> Valid Out/1
  Mux/1 -> Data Out/1
  Constant1/1 -> Mux/3
  Constant/1 -> Mux/2

== system qpsk_rx_frame_sync/Frame Synchronisation/Frame Sync/DQPSK Imag Decision ==
  Data In : Inport
  Valid In : Inport  Port=2
  Logical1 : xbsIndex_r4/Logical  logical_function=XOR  inputs=2  en=off  latency=0  precision=Full  arith_type=Unsigned  n_bits=16  bin_pt=0  align_bp=on  dbl_ovrd=off  block_type=logical
  Register : xbsIndex_r4/Register  init=0  rst=off  en=on  dbl_ovrd=off  block_type=register
  Register2 : xbsIndex_r4/Register  init=0  rst=off  en=off  dbl_ovrd=off  block_type=register
  Register3 : xbsIndex_r4/Register  init=0  rst=off  en=on  dbl_ovrd=off  block_type=register
  Register4 : xbsIndex_r4/Register  init=0  rst=off  en=on  dbl_ovrd=off  block_type=register
  Register5 : xbsIndex_r4/Register  init=0  rst=off  en=off  dbl_ovrd=off  block_type=register
  Data Out : Outport  VectorParamsAs1DForOutWhenUnconnected=off
  Valid Out : Outport  Port=2  VectorParamsAs1DForOutWhenUnconnected=off
  wires:
  Data In/1 -> Register/1
  Register5/1 -> Valid Out/1
  Valid In/1 -> Register/2, Register2/1
  Register3/1 -> Logical1/1
  Register/1 -> Register3/1, Logical1/2
  Logical1/1 -> Register4/1
  Register2/1 -> Register3/2, Register5/1, Register4/2
  Register4/1 -> Data Out/1

== system qpsk_rx_frame_sync/Frame Synchronisation/Frame Sync/DQPSK Real Convert ==
  Data In : Inport
  Valid In : Inport  Port=2
  Constant : xbsIndex_r4/Constant  const=1.0  gui_display_data_type=Fixed-point  arith_type=Signed (2's comp)  n_bits=2  bin_pt=0  preci_type=Single  exp_width=8  frac_width=24  explicit_period=off  period=1  equ=P=C  opselect=C  inp2=PCIN>>17  opr=+  inp1=P  carry=CIN  dbl_ovrd=off  block_type=constant
  Constant1 : xbsIndex_r4/Constant  const=-1.0  gui_display_data_type=Fixed-point  arith_type=Signed (2's comp)  n_bits=2  bin_pt=0  preci_type=Single  exp_width=8  frac_width=24  explicit_period=off  period=1  equ=P=C  opselect=C  inp2=PCIN>>17  opr=+  inp1=P  carry=CIN  dbl_ovrd=off  block_type=constant
  Mux : xbsIndex_r4/Mux  inputs=2  en=off  latency=0  precision=Full  arith_type=Unsigned  n_bits=16  bin_pt=14  quantization=Truncate  overflow=Wrap  dbl_ovrd=off  block_type=mux
  Data Out : Outport  VectorParamsAs1DForOutWhenUnconnected=off
  Valid Out : Outport  Port=2  VectorParamsAs1DForOutWhenUnconnected=off
  wires:
  Constant/1 -> Mux/2
  Constant1/1 -> Mux/3
  Mux/1 -> Data Out/1
  Valid In/1 -> Valid Out/1
  Data In/1 -> Mux/1

== system qpsk_rx_frame_sync/Frame Synchronisation/Frame Sync/DQPSK Real Decision ==
  Data In : Inport
  Valid In : Inport  Port=2
  Logical1 : xbsIndex_r4/Logical  logical_function=XOR  inputs=2  en=off  latency=0  precision=Full  arith_type=Unsigned  n_bits=16  bin_pt=0  align_bp=on  dbl_ovrd=off  block_type=logical
  Register : xbsIndex_r4/Register  init=0  rst=off  en=on  dbl_ovrd=off  block_type=register
  Register2 : xbsIndex_r4/Register  init=0  rst=off  en=off  dbl_ovrd=off  block_type=register
  Register3 : xbsIndex_r4/Register  init=0  rst=off  en=on  dbl_ovrd=off  block_type=register
  Register4 : xbsIndex_r4/Register  init=0  rst=off  en=on  dbl_ovrd=off  block_type=register
  Register5 : xbsIndex_r4/Register  init=0  rst=off  en=off  dbl_ovrd=off  block_type=register
  Data Out : Outport  VectorParamsAs1DForOutWhenUnconnected=off
  Valid Out : Outport  Port=2  VectorParamsAs1DForOutWhenUnconnected=off
  wires:
  Register4/1 -> Data Out/1
  Register2/1 -> Register4/2, Register5/1, Register3/2
  Logical1/1 -> Register4/1
  Register/1 -> Logical1/2, Register3/1
  Register3/1 -> Logical1/1
  Valid In/1 -> Register2/1, Register/2
  Register5/1 -> Valid Out/1
  Data In/1 -> Register/1

== system qpsk_rx_frame_sync/Frame Synchronisation/Frame Sync/Rising Edge Detector ==
  Input : Inport
  Inverter : xbsIndex_r4/Inverter  en=off  latency=0  dbl_ovrd=off  block_type=inv
  Logical1 : xbsIndex_r4/Logical  logical_function=AND  inputs=2  en=off  latency=0  precision=Full  arith_type=Unsigned  n_bits=16  bin_pt=0  align_bp=on  dbl_ovrd=off  block_type=logical
  Register2 : xbsIndex_r4/Register  init=0  rst=off  en=off  dbl_ovrd=off  block_type=register
  Output : Outport  VectorParamsAs1DForOutWhenUnconnected=off
  wires:
  Logical1/1 -> Output/1
  Input/1 -> Logical1/2, Register2/1
  Inverter/1 -> Logical1/1
  Register2/1 -> Inverter/1

== system qpsk_rx_frame_sync/Frame Synchronisation/Frame Sync/Shift Register ==
  Data In : Inport
  Valid In : Inport  Port=2
  Concat : xbsIndex_r4/Concat  num_inputs=4  dbl_ovrd=off  block_type=concat
  Constant : xbsIndex_r4/Constant  const=4  gui_display_data_type=Fixed-point  arith_type=Unsigned  n_bits=3  bin_pt=0  preci_type=Single  exp_width=8  frac_width=24  explicit_period=off  period=1  equ=P=C  opselect=C  inp2=PCIN>>17  opr=+  inp1=P  carry=CIN  dbl_ovrd=off  block_type=constant
  Counter : xbsIndex_r4/Counter  cnt_type=Count Limited  cnt_to=4  operation=Up  start_count=0  cnt_by_val=1  arith_type=Unsigned  n_bits=3  bin_pt=0  load_pin=off  rst=on  en=on  explicit_period=off  period=1  use_behavioral_HDL=off  implementation=Fabric  dbl_ovrd=off  block_type=counter
  Register{4..7} (4 alike) : xbsIndex_r4/Register  init=0  rst=off  en=on  dbl_ovrd=off  block_type=register
  Relational : xbsIndex_r4/Relational  mode=a=b  op_type=Bool  en=off  latency=0  dbl_ovrd=off  block_type=relational
  Data Out : Outport  VectorParamsAs1DForOutWhenUnconnected=off
  Valid Out : Outport  Port=2  VectorParamsAs1DForOutWhenUnconnected=off
  wires:
  Relational/1 -> Valid Out/1, Counter/1
  Constant/1 -> Relational/2
  Counter/1 -> Relational/1
  Concat/1 -> Data Out/1
  Data In/1 -> Register7/1
  Register5/1 -> Register4/1, Concat/3
  Register4/1 -> Concat/4
  Register7/1 -> Register6/1, Concat/1
  Register6/1 -> Register5/1, Concat/2
  Valid In/1 -> Register7/2, Register4/2, Register5/2, Register6/2, Counter/2

== system qpsk_rx_frame_sync/QPSK System/QPSK RX Generation/RRC Receive Filter ==
  Data In : Inport
  Data Type Conversion2 : DataTypeConversion  OutDataTypeStr=fixdt(1,16,14)
  FDATool : xbsIndex_r4/FDATool  block_type=fdatool
      settings: infoedit=FDATool
  FIR Decimation : dspmlti4/FIR Decimation  FilterSource=Dialog parameters  h=xlfda_numerator('FDATool')  D=4  filtStruct=Direct form  FilterObject=FDECIM  framing=Allow multirate processing  inputOffset=0  outputBufInitCond=0  roundingMode=Floor  overflowMode=off  firstCoeffMode=Binary point scaling  firstCoeffWordLength=16  firstCoeffFracLength=14  firstCoeffDataTypeStr=fixdt(1,16,14)  firstCoeffMin=[]  firstCoeffMax=[]  firstCoeffLastDataTypeStr=fixdt(1,16,14)  outputDataTypeStr=Inherit: Same as accumulator  outputMin=[]  outputMax=[]  outputLastDataTypeStr=Inherit: Same as accumulator
  Data Out : Outport  VectorParamsAs1DForOutWhenUnconnected=off
  wires:
  Data Type Conversion2/1 -> Data Out/1
  Data In/1 -> FIR Decimation/1
  FIR Decimation/1 -> Data Type Conversion2/1

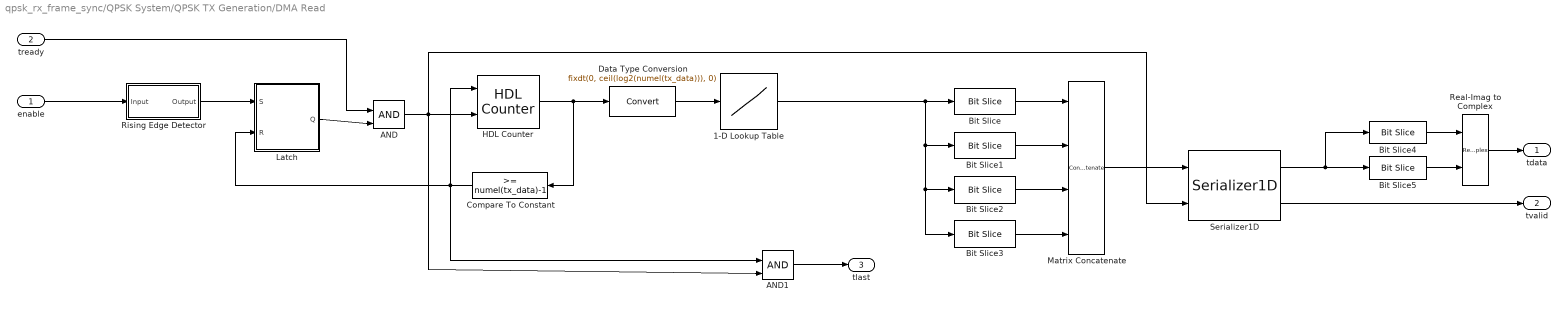
== system qpsk_rx_frame_sync/QPSK System/QPSK TX Generation/DMA Read ==
  enable : Inport
  tready : Inport  Port=2
  1-D Lookup Table : Lookup_n-D  NumberOfTableDimensions=1  BreakpointsForDimension1=[0:1:numel(tx_data)-1]  Table=tx_data  TableDataTypeStr=Inherit: Inherit from 'Table data'  ExtrapMethod=Clip  InternalRulePriority=Speed  OutDataTypeStr=Inherit: Inherit from 'Table data'  RndMeth=Simplest  InputSameDT=on
  AND : Logic  IconShape=distinctive  AllPortsSameDT=off  OutDataTypeStr=boolean
  AND1 : Logic  IconShape=distinctive  AllPortsSameDT=off  OutDataTypeStr=boolean
  Bit Slice : hdlsllib/Logic and Bit Operations/Bit Slice  lidx=1  ridx=0
      settings: SourceProductBaseCode=SL
  Bit Slice1 : hdlsllib/Logic and Bit Operations/Bit Slice  lidx=3  ridx=2
      settings: SourceProductBaseCode=SL
  Bit Slice2 : hdlsllib/Logic and Bit Operations/Bit Slice  lidx=5  ridx=4
      settings: SourceProductBaseCode=SL
  Bit Slice3 : hdlsllib/Logic and Bit Operations/Bit Slice  lidx=7  ridx=6
      settings: SourceProductBaseCode=SL
  Bit Slice4 : hdlsllib/Logic and Bit Operations/Bit Slice  lidx=0  ridx=0
      settings: SourceProductBaseCode=SL
  Bit Slice5 : hdlsllib/Logic and Bit Operations/Bit Slice  lidx=1  ridx=1
      settings: SourceProductBaseCode=SL
  Compare To Constant : simulink/Logic and Bit Operations/Compare To Constant  relop=>=  const=numel(tx_data)-1  OutDataTypeStr=boolean
  Data Type Conversion : DataTypeConversion  OutDataTypeStr=fixdt(0, ceil(log2(numel(tx_data))), 0)
  HDL Counter : hdlsllib/Sources/HDL Counter  CountType=Free running  CountInit=0  CountStep=1  CountMax=25  CountFromType=Initial value  CountFrom=0  CountResetPort=on  CountLoadPort=off  CountEnbPort=on  CountDirPort=off  CountDataType=Unsigned  CountWordLen=32  CountFracLen=0  CountSampTime=1
  Latch : Subsystem
  Matrix Concatenate : Concatenate  NumInputs=4  Mode=Multidimensional array  ConcatenateDimension=2
  Real-Imag to Complex : RealImagToComplex
  Rising Edge Detector : Subsystem
  Serializer1D : hdlsllib/HDL Operations/Serializer1D  Ratio=4  IdleCycles=0  validIn=on  startOut=off  validOut=on  inputDataDimensions=-1  inputSampleTime=-1  inputSignalType=auto
      settings: SourceProductBaseCode=SL
  tdata : Outport  VectorParamsAs1DForOutWhenUnconnected=off
  tvalid : Outport  Port=2  VectorParamsAs1DForOutWhenUnconnected=off
  tlast : Outport  Port=3  VectorParamsAs1DForOutWhenUnconnected=off
  wires:
  Serializer1D/1 -> Bit Slice4/1, Bit Slice5/1
  Real-Imag to Complex/1 -> tdata/1
  Bit Slice5/1 -> Real-Imag to Complex/2
  Bit Slice4/1 -> Real-Imag to Complex/1
  AND1/1 -> tlast/1
  tready/1 -> AND/1
  Latch/1(Q) -> AND/2
  AND/1 -> HDL Counter/2, Serializer1D/2, AND1/2
  Rising Edge Detector/1(Output) -> Latch/1(S)
  Data Type Conversion/1 -> 1-D Lookup Table/1
  HDL Counter/1 -> Data Type Conversion/1, Compare To Constant/1
  enable/1 -> Rising Edge Detector/1(Input)
  Compare To Constant/1 -> Latch/2(R), HDL Counter/1, AND1/1
  Matrix Concatenate/1 -> Serializer1D/1
  Bit Slice/1 -> Matrix Concatenate/1
  Bit Slice3/1 -> Matrix Concatenate/4
  Bit Slice1/1 -> Matrix Concatenate/2
  Bit Slice2/1 -> Matrix Concatenate/3
  1-D Lookup Table/1 -> Bit Slice3/1, Bit Slice2/1, Bit Slice1/1, Bit Slice/1
  Serializer1D/2 -> tvalid/1

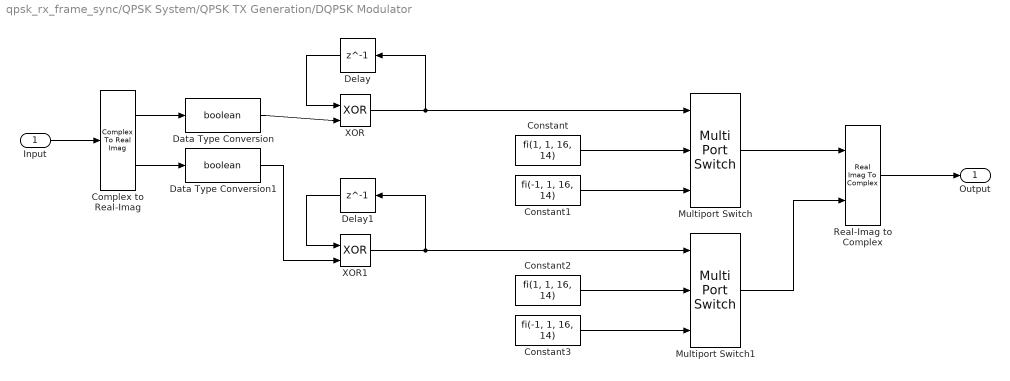
== system qpsk_rx_frame_sync/QPSK System/QPSK TX Generation/DQPSK Modulator ==
  Input : Inport
  Complex to Real-Imag : ComplexToRealImag
  Constant : Constant  Value=fi(1, 1, 16, 14)  OutDataTypeStr=fixdt(1,16,14)  SampleTime=-1
  Constant1 : Constant  Value=fi(-1, 1, 16, 14)  OutDataTypeStr=fixdt(1,16,14)  SampleTime=-1
  Constant2 : Constant  Value=fi(1, 1, 16, 14)  OutDataTypeStr=fixdt(1,16,14)  SampleTime=-1
  Constant3 : Constant  Value=fi(-1, 1, 16, 14)  OutDataTypeStr=fixdt(1,16,14)  SampleTime=-1
  Data Type Conversion : DataTypeConversion  OutDataTypeStr=boolean  RndMeth=Round
  Data Type Conversion1 : DataTypeConversion  OutDataTypeStr=boolean  RndMeth=Round
  Delay : Delay  DelayLength=1
  Delay1 : Delay  DelayLength=1
  Multiport Switch : MultiPortSwitch  DataPortOrder=Zero-based contiguous  Inputs=2  zeroidx=on
  Multiport Switch1 : MultiPortSwitch  DataPortOrder=Zero-based contiguous  Inputs=2  zeroidx=on
  Real-Imag to Complex : RealImagToComplex
  XOR : Logic  Operator=XOR  IconShape=distinctive  AllPortsSameDT=off  OutDataTypeStr=boolean
  XOR1 : Logic  Operator=XOR  IconShape=distinctive  AllPortsSameDT=off  OutDataTypeStr=boolean
  Output : Outport  VectorParamsAs1DForOutWhenUnconnected=off
  wires:
  Data Type Conversion1/1 -> XOR1/2
  Data Type Conversion/1 -> XOR/2
  Multiport Switch1/1 -> Real-Imag to Complex/2
  Constant3/1 -> Multiport Switch1/3
  Constant2/1 -> Multiport Switch1/2
  Delay1/1 -> XOR1/1
  XOR1/1 -> Multiport Switch1/1, Delay1/1
  Complex to Real-Imag/2 -> Data Type Conversion1/1
  Input/1 -> Complex to Real-Imag/1
  Complex to Real-Imag/1 -> Data Type Conversion/1
  XOR/1 -> Delay/1, Multiport Switch/1
  Delay/1 -> XOR/1
  Constant/1 -> Multiport Switch/2
  Constant1/1 -> Multiport Switch/3
  Multiport Switch/1 -> Real-Imag to Complex/1
  Real-Imag to Complex/1 -> Output/1
